simulink subsystem "Actuator"  (R2023a)
settings: Solver=VariableStepAuto  StartTime=0.0  StopTime=10.0  RelTol=1e-3
undefined symbols (not defined in the file): DemoControllers
settings Model: Creator=Maxim Kozlov  LastModifiedBy=Maxim

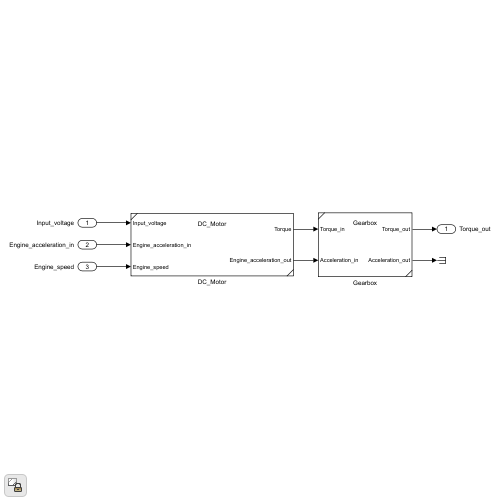
[thumbnail: Simulink's stored preview of the top-level diagram]
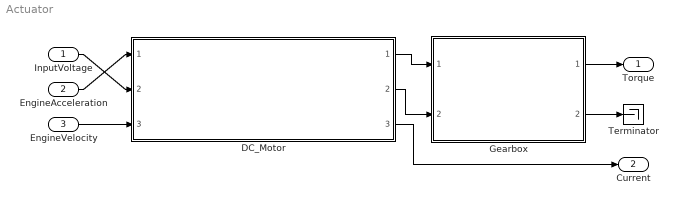
== system Actuator ==
  InputVoltage : Inport
  EngineAcceleration : Inport  Port=2
  EngineVelocity : Inport  Port=3
  DC_Motor : Subsystem  ReferencedSubsystem=DC_Motor  Km=DemoControllers.DCMotor.Km  Kw=DemoControllers.DCMotor.Kw  R=DemoControllers.DCMotor.R  L=DemoControllers.DCMotor.L  J_engine=DemoControllers.DCMotor.J
  Gearbox : Subsystem  ReferencedSubsystem=Gearbox  i=DemoControllers.Reductor.i  J=DemoControllers.Reductor.J
  Terminator : Terminator
  Torque : Outport
  Current : Outport  Port=2
  wires:
  EngineAcceleration/1 -> DC_Motor/1
  EngineVelocity/1 -> DC_Motor/3
  DC_Motor/1 -> Gearbox/1
  InputVoltage/1 -> DC_Motor/2
  DC_Motor/2 -> Gearbox/2
  Gearbox/1 -> Torque/1
  Gearbox/2 -> Terminator/1
  DC_Motor/3 -> Current/1
